simulink model "Gyro_Outage_Unit_Test"  (R2018b)
settings: Solver=VariableStepAuto  StartTime=0.0  StopTime=5600  FixedStep=fswParams.sample_time_s  RelTol=1e-8  AbsTol=1e-8
undefined symbols (not defined in the file or in its folder): B_eci_unit, Conversion_lib, DiscIntNeverNeededParam, e2sun_eci_unit, ECLIPSE, env_acc_mps2, Environment_lib, fswParams, gyro_body_radps, gyro_meas_valid, mag_body_T, mag_meas_valid, MEKF_Conversion_lib, MEKF_lib, photodiodes_A, q_body, r_eci_km, satelliteDynamics_lib, sc2sun_eci_unit, Sensors_Lib, simParams, solar_panel_power_W, sun_sensor_lib, sunsensor_2body_lib, sunsensor_body_deg, sunsensor_body_rad, sunsensor_valid, Triad, Triad_lib, v_eci_km, w_body_radps
libraries: aerolibutil x11, vrlib x10, sharedutil x8, simulink x5, dspmathops x4, sharedtransform x3, magnetometer_lib x3, gyroscope_lib x2, gravityGrad_Lib x1, atmoDrag_lib x1, magField_lib x1, solarPressure_lib x1
(part 1 of 3)
settings Model: Creator=kylle  LastModifiedBy=kylle

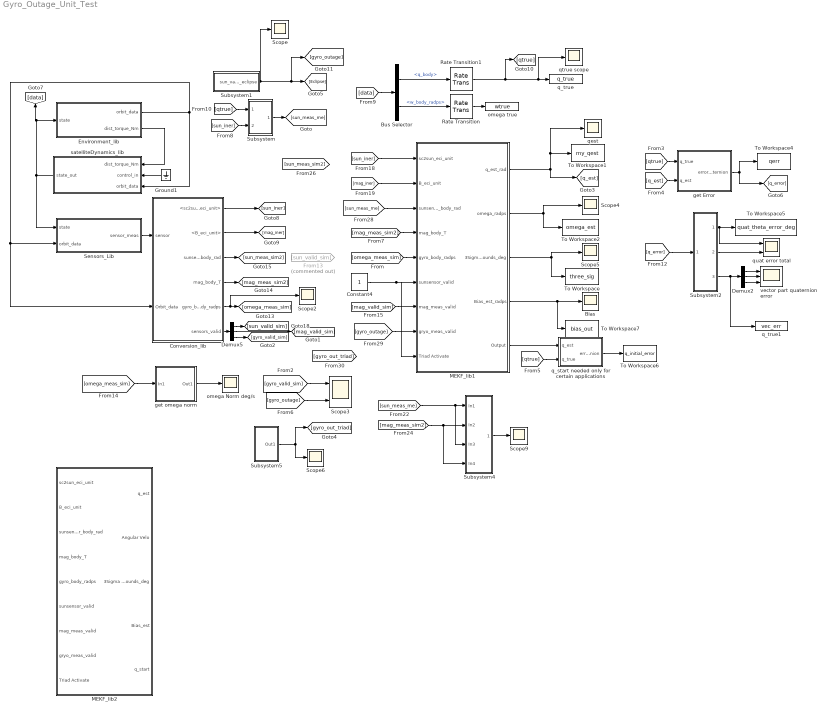
== system Gyro_Outage_Unit_Test ==
  Bias : Scope
  Bus Selector : BusSelector  OutputSignals=q_body,w_body_radps
  Constant4 : Constant
  Conversion_lib : Subsystem  AncestorBlock=MEKF_Conversion_lib/Conversion_lib
  Demux2 : Demux  Outputs=3
  Demux5 : Demux  Outputs=3
  Environment_lib : Subsystem  AncestorBlock=Environment_lib/Environment_lib
  From13 : From  Commented=on  GotoTag=sun_valid_sim
  Ground1 : Ground
  MEKF_lib1 : Subsystem  AncestorBlock=MEKF_lib/MEKF_lib
  MEKF_lib2 : Subsystem  AncestorBlock=MEKF_lib/MEKF_lib
  Rate Transition : RateTransition  InitialCondition=[0;0;0]  OutPortSampleTime=fswParams.sample_time_s
  Rate Transition1 : RateTransition  InitialCondition=[1;0;0;0]  OutPortSampleTime=fswParams.sample_time_s
  Scope{,2,4..6,9} (6 alike) : Scope
  Scope3 : Scope  NumInputPorts=2
  Sensors_Lib : Subsystem  AncestorBlock=Sensors_Lib/Sensors_Lib
  Subsystem : Subsystem
  Subsystem1 : Subsystem
  Subsystem2 : Subsystem
  Subsystem4 : Subsystem
  Subsystem5 : Subsystem
  To Workspace : ToWorkspace  VariableName=three_sig  SaveFormat=Timeseries  SampleTime=-1
  To Workspace1 : ToWorkspace  VariableName=my_qest  SaveFormat=Timeseries  SampleTime=-1
  To Workspace2 : ToWorkspace  VariableName=omega_est  SaveFormat=Timeseries  SampleTime=-1
  To Workspace4 : ToWorkspace  VariableName=qerr  SaveFormat=Timeseries  SampleTime=-1
  To Workspace5 : ToWorkspace  VariableName=quat_theta_error_deg  SaveFormat=Timeseries  SampleTime=-1
  To Workspace6 : ToWorkspace  VariableName=q_initial_error  SaveFormat=Timeseries  SampleTime=-1
  To Workspace7 : ToWorkspace  VariableName=bias_out  SaveFormat=Timeseries  SampleTime=-1
  get Error : Subsystem
  get omega norm : Subsystem
  omega Norm deg/s : Scope
  omega true : ToWorkspace  VariableName=wtrue  SaveFormat=Timeseries  SampleTime=-1
  q_start needed only for certain applications : Subsystem
  q_true : ToWorkspace  VariableName=q_true  SaveFormat=Timeseries  SampleTime=-1
  q_true1 : ToWorkspace  VariableName=vec_err  SaveFormat=Timeseries  SampleTime=-1
  qest : Scope
  "qtrue scope " : Scope
  quat error total : Scope  NumInputPorts=2
  satelliteDynamics_lib : Subsystem  AncestorBlock=satelliteDynamics_lib/satelliteDynamics_lib
  vector part quaternion error : Scope  NumInputPorts=3
  wires:
  get Error/1(error_quaternion) -> To Workspace4/1, [q_error]
  [q_est] -> get Error/2(q_est)
  [qtrue] -> get Error/1(q_true)
  Demux2/1 -> vector part quaternion error/1
  Demux2/2 -> vector part quaternion error/2
  Demux2/3 -> vector part quaternion error/3
  MEKF_lib1/1(q_est_rad) -> [q_est], qest/1, To Workspace1/1
  MEKF_lib1/2(omega_radps) -> To Workspace2/1, Scope4/1
  MEKF_lib1/3("3Sigma Bounds_deg ") -> Scope5/1, To Workspace/1
  MEKF_lib1/4(Bias_est_radps) -> Bias/1, To Workspace7/1
  Ground1/1 -> satelliteDynamics_lib/2(control_in)
  Environment_lib/1(orbit_data) -> satelliteDynamics_lib/3(orbit_data), Sensors_Lib/2(orbit_data), Conversion_lib/2(Orbit_data)
  Environment_lib/2(dist_torque_Nm) -> satelliteDynamics_lib/1(dist_torque_Nm)
  satelliteDynamics_lib/1(state_out) -> Environment_lib/1(state), [data], Sensors_Lib/1(state)
  Bus Selector/2 -> Rate Transition/1  "<w_body_radps>"
  [data] -> Bus Selector/1
  Bus Selector/1 -> Rate Transition1/1  "<q_body>"
  Sensors_Lib/1(sensor_meas) -> Conversion_lib/1(sensor)
  [mag_meas_sim2] -> MEKF_lib1/4(mag_body_T)
  [sun_iner] -> MEKF_lib1/1(sc2sun_eci_unit)
  [mag_iner] -> MEKF_lib1/2(B_eci_unit)
  [gyro_valid_sim] -> Scope3/1
  Conversion_lib/2(<B_eci_unit>) -> [mag_iner]
  Conversion_lib/1(<sc2sun_eci_unit>) -> [sun_iner]
  Conversion_lib/4(mag_body_T) -> [mag_meas_sim2]
  Conversion_lib/5(gyro_body_radps) -> Scope2/1, [omega_meas_sim]
  Demux5/2 -> [mag_valid_sim]
  Demux5/3 -> [gyro_valid_sim]
  Conversion_lib/6("sensors_valid ") -> Demux5/1
  q_start needed only for certain applications/1(error_quaternion) -> To Workspace6/1
  [qtrue] -> q_start needed only for certain applications/2(q_true)
  [qtrue] -> Subsystem/1(In1)
  [sun_iner] -> Subsystem/2(In2)
  Subsystem/1(Out1) -> [sun_meas_me]
  Conversion_lib/3(sunsensor_body_rad) -> [sun_meas_sim2]
  Demux5/1 -> [sun_valid_sim]
  Subsystem2/1(Out1) -> quat error total/1, To Workspace5/1
  [q_error] -> Subsystem2/1(In1)
  Subsystem2/2(Out2) -> quat error total/2
  Subsystem2/3(Out3) -> q_true1/1, Demux2/1
  Subsystem1/1(sun_valid_eclipse) -> Scope/1, [Eclipse], [gyro_outage]
  [omega_meas_sim] -> MEKF_lib1/5(gyro_body_radps)
  [mag_valid_sim] -> MEKF_lib1/7(mag_meas_valid)
  Rate Transition/1 -> omega true/1
  Rate Transition1/1 -> "qtrue scope "/1, q_true/1, [qtrue]
  [omega_meas_sim] -> get omega norm/1(In1)
  get omega norm/1(Out1) -> omega Norm deg/s/1
  [sun_meas_me] -> Subsystem4/3(In3), Subsystem4/1(In1)
  [mag_meas_sim2] -> Subsystem4/4(In4), Subsystem4/2(In2)
  Subsystem4/1(Out1) -> Scope9/1
  [sun_meas_me] -> MEKF_lib1/3(sunsensor_body_rad)
  Constant4/1 -> MEKF_lib1/9(Triad Activate), MEKF_lib1/6(sunsensor_valid)
  Subsystem5/1(Out1) -> [gyro_out_triad], Scope6/1
  [gyro_outage] -> MEKF_lib1/8(gryo_meas_valid)
  [gyro_outage] -> Scope3/2
  MEKF_lib1/5(Output) -> q_start needed only for certain applications/1(q_est)

== system Gyro_Outage_Unit_Test/Conversion_lib ==
  sensor : Inport
  Orbit_data : Inport  Port=2
  Bus Selector1 : BusSelector  OutputSignals=sc2sun_eci_unit,B_eci_unit
  Bus Selector2 : BusSelector  OutputSignals=sunsensor_body_deg,mag_body_T,gyro_body_radps,sunsensor_valid,mag_meas_valid,gyro_meas_valid
  Mux : Mux  Inputs=3
  Variable Selector : S-Function  AncestorBlock=dspindex/Variable Selector  FunctionName=sdspperm2  Parameters=1,NumInputs, rowsOrCols, IdxMode, Elements, FillMode, FillValues, errmode, 0, ZerOneIdxMode  SFunctionDeploymentMode=off  EnableBusSupport=off  mask(Variable Selector){NumInputs=1, rowsOrCols=Columns, IdxMode=Fixed, Elements=[1], ZerOneIdxMode=One-based, errmode=Clip Index, FillMode=off, FillValues=0, ShowPortLabels=off}
      mask prompts: NumInputs "Number of input signals:"; rowsOrCols "Select:"; IdxMode "Selector mode:"; ZerOneIdxMode "Index mode:"; errmode "Invalid index:"; FillMode "Fill empty spaces in outputs (for logical indexing)"; FillValues "Fill values:"; ShowPortLabels "Unused:"
      mask help:
      | Selects and/or reorders the rows or columns of the input according to a specified vector of indices (the indices need not be unique). The 'Selector mode' parameter determines whether the block uses the same indices for every input ('Fixed'), or uses different indices for every input ('Variable'). When set to 'Variable', you provide the vector of indices through an input port.
      |
      | When the indices are of Boolean data type the block performs logical indexing.
      mask init:
      | if ~isempty(NumInputs) && isfinite(NumInputs) && ~isnan(NumInputs) ...
      |  && isscalar(NumInputs) && isreal(NumInputs) && (NumInputs>0)
      |     maskdisplay = ['disp([''Select\n' get_param(gcbh, 'rowsOrCols') ''']);'];
      | 
      |     for i=1:NumInputs
      |         istr = int2str(i);
      |         maskdisplay = [maskdisplay 'port_label(''input'',' istr, ',''In' istr ''');'];
      |         maskdisplay = [maskdisplay 'port_label(''output'',' istr, ',''Out' istr ''');'];
      |     end
      | 
      |     if  IdxMode==2
      |         istr = int2str(NumInputs+1);
      |         maskdisplay = [maskdisplay 'port_label(''input'',' istr, ',''Idx'');'];
      |     end
      |     set_param(gcb, 'MaskDisplay', maskdisplay);
      | end
      mask Help: eval('blocksethelp');
      mask TypeOptions rowsOrCols: Rows | Columns
      mask TypeOptions IdxMode: Fixed | Variable
      mask Callback IdxMode: dspblkperm2;
      mask TypeOptions ZerOneIdxMode: Zero-based | One-based
      mask TypeOptions errmode: Clip Index | Clip and Warn | Generate Error
      mask Callback FillMode: dspblkperm2;
      mask Display: disp(['Select\nColumns']);port_label('input',1,'In1');port_label('output',1,'Out1');
  Variable Selector1 : S-Function  AncestorBlock=dspindex/Variable Selector  FunctionName=sdspperm2  Parameters=1,NumInputs, rowsOrCols, IdxMode, Elements, FillMode, FillValues, errmode, 0, ZerOneIdxMode  SFunctionDeploymentMode=off  EnableBusSupport=off  mask(Variable Selector){NumInputs=1, rowsOrCols=Columns, IdxMode=Fixed, Elements=[1], ZerOneIdxMode=One-based, errmode=Clip Index, FillMode=off, FillValues=0, ShowPortLabels=off}
      mask prompts: NumInputs "Number of input signals:"; rowsOrCols "Select:"; IdxMode "Selector mode:"; ZerOneIdxMode "Index mode:"; errmode "Invalid index:"; FillMode "Fill empty spaces in outputs (for logical indexing)"; FillValues "Fill values:"; ShowPortLabels "Unused:"
      mask help:
      | Selects and/or reorders the rows or columns of the input according to a specified vector of indices (the indices need not be unique). The 'Selector mode' parameter determines whether the block uses the same indices for every input ('Fixed'), or uses different indices for every input ('Variable'). When set to 'Variable', you provide the vector of indices through an input port.
      |
      | When the indices are of Boolean data type the block performs logical indexing.
      mask init: same as Gyro_Outage_Unit_Test/Conversion_lib/Variable Selector
      mask Help: eval('blocksethelp');
      mask TypeOptions rowsOrCols: Rows | Columns
      mask TypeOptions IdxMode: Fixed | Variable
      mask Callback IdxMode: dspblkperm2;
      mask TypeOptions ZerOneIdxMode: Zero-based | One-based
      mask TypeOptions errmode: Clip Index | Clip and Warn | Generate Error
      mask Callback FillMode: dspblkperm2;
      mask Display: disp(['Select\nColumns']);port_label('input',1,'In1');port_label('output',1,'Out1');
  Variable Selector2 : S-Function  AncestorBlock=dspindex/Variable Selector  FunctionName=sdspperm2  Parameters=1,NumInputs, rowsOrCols, IdxMode, Elements, FillMode, FillValues, errmode, 0, ZerOneIdxMode  SFunctionDeploymentMode=off  EnableBusSupport=off  mask(Variable Selector){NumInputs=1, rowsOrCols=Rows, IdxMode=Fixed, Elements=[1], ZerOneIdxMode=One-based, errmode=Clip Index, FillMode=off, FillValues=0, ShowPortLabels=off}
      mask prompts: NumInputs "Number of input signals:"; rowsOrCols "Select:"; IdxMode "Selector mode:"; ZerOneIdxMode "Index mode:"; errmode "Invalid index:"; FillMode "Fill empty spaces in outputs (for logical indexing)"; FillValues "Fill values:"; ShowPortLabels "Unused:"
      mask help:
      | Selects and/or reorders the rows or columns of the input according to a specified vector of indices (the indices need not be unique). The 'Selector mode' parameter determines whether the block uses the same indices for every input ('Fixed'), or uses different indices for every input ('Variable'). When set to 'Variable', you provide the vector of indices through an input port.
      |
      | When the indices are of Boolean data type the block performs logical indexing.
      mask init: same as Gyro_Outage_Unit_Test/Conversion_lib/Variable Selector
      mask Help: eval('blocksethelp');
      mask TypeOptions rowsOrCols: Rows | Columns
      mask TypeOptions IdxMode: Fixed | Variable
      mask Callback IdxMode: dspblkperm2;
      mask TypeOptions ZerOneIdxMode: Zero-based | One-based
      mask TypeOptions errmode: Clip Index | Clip and Warn | Generate Error
      mask Callback FillMode: dspblkperm2;
      mask Display: disp(['Select\nRows']);port_label('input',1,'In1');port_label('output',1,'Out1');
  Variable Selector3 : S-Function  AncestorBlock=dspindex/Variable Selector  FunctionName=sdspperm2  Parameters=1,NumInputs, rowsOrCols, IdxMode, Elements, FillMode, FillValues, errmode, 0, ZerOneIdxMode  SFunctionDeploymentMode=off  EnableBusSupport=off  mask(Variable Selector){NumInputs=1, rowsOrCols=Rows, IdxMode=Fixed, Elements=[1], ZerOneIdxMode=One-based, errmode=Clip Index, FillMode=off, FillValues=0, ShowPortLabels=off}
      mask prompts: NumInputs "Number of input signals:"; rowsOrCols "Select:"; IdxMode "Selector mode:"; ZerOneIdxMode "Index mode:"; errmode "Invalid index:"; FillMode "Fill empty spaces in outputs (for logical indexing)"; FillValues "Fill values:"; ShowPortLabels "Unused:"
      mask help:
      | Selects and/or reorders the rows or columns of the input according to a specified vector of indices (the indices need not be unique). The 'Selector mode' parameter determines whether the block uses the same indices for every input ('Fixed'), or uses different indices for every input ('Variable'). When set to 'Variable', you provide the vector of indices through an input port.
      |
      | When the indices are of Boolean data type the block performs logical indexing.
      mask init: same as Gyro_Outage_Unit_Test/Conversion_lib/Variable Selector
      mask Help: eval('blocksethelp');
      mask TypeOptions rowsOrCols: Rows | Columns
      mask TypeOptions IdxMode: Fixed | Variable
      mask Callback IdxMode: dspblkperm2;
      mask TypeOptions ZerOneIdxMode: Zero-based | One-based
      mask TypeOptions errmode: Clip Index | Clip and Warn | Generate Error
      mask Callback FillMode: dspblkperm2;
      mask Display: disp(['Select\nRows']);port_label('input',1,'In1');port_label('output',1,'Out1');
  sunsensor_body_rad1 : Subsystem  AncestorBlock=sunsensor_2body_lib/sunsensor_body_rad
  <sc2sun_eci_unit> : Outport
  <B_eci_unit> : Outport  Port=2
  sunsensor_body_rad : Outport  Port=3
  mag_body_T : Outport  Port=4
  gyro_body_radps : Outport  Port=5
  "sensors_valid " : Outport  Port=6
  wires:
  Bus Selector2/3 -> Variable Selector/1  "<gyro_body_radps>"
  Bus Selector1/2 -> <B_eci_unit>/1  "<B_eci_unit>"
  Bus Selector2/1 -> sunsensor_body_rad1/1(<sunsensor_body_deg>)  "<sunsensor_body_deg>"
  Bus Selector2/2 -> Variable Selector1/1  "<mag_body_T>"
  sunsensor_body_rad1/1(Out1) -> sunsensor_body_rad/1
  Bus Selector2/5 -> Variable Selector3/1  "<mag_meas_valid>"
  Bus Selector2/6 -> Variable Selector2/1  "<gyro_meas_valid>"
  sensor/1 -> Bus Selector2/1
  Variable Selector1/1 -> mag_body_T/1
  Bus Selector1/1 -> <sc2sun_eci_unit>/1  "<sc2sun_eci_unit>"
  Orbit_data/1 -> Bus Selector1/1
  Variable Selector/1 -> gyro_body_radps/1
  Variable Selector2/1 -> Mux/3
  Variable Selector3/1 -> Mux/2
  Bus Selector2/4 -> Mux/1  "<sunsensor_valid>"
  Mux/1 -> "sensors_valid "/1

== system Gyro_Outage_Unit_Test/Environment_lib ==
  state : Inport
  Bus Assignment : BusAssignment  AssignedSignals=env_acc_mps2,e2sun_eci_unit,sc2sun_eci_unit,ECLIPSE,B_eci_unit
  Disturbances : Subsystem
  Terminator{1..2,5,8..9,11..16} (11 alike) : Terminator
  clock_lib : clock_lib/clock_lib  SystemSampleTime=-1
  orbit_data_bus : orbit_data_bus/orbit_data_bus  SystemSampleTime=-1
  "time_lib " : time_Lib/time_lib    SystemSampleTime=-1
  orbit_data : Outport
  dist_torque_Nm : Outport  Port=2
  wires:
  Bus Assignment/1 -> orbit_data/1
  orbit_data_bus/1 -> Bus Assignment/1
  "time_lib "/10 -> Terminator2/1
  state/1 -> Disturbances/1(state)
  Disturbances/1(env_acc_mps2) -> Bus Assignment/2
  Disturbances/4(ECLIPSE) -> Bus Assignment/5
  "time_lib "/9 -> Terminator13/1
  [ymdhms_utc] -> Disturbances/5(ymdhms_utc)
  "time_lib "/7 -> Terminator11/1
  "time_lib "/11 -> Terminator14/1
  "time_lib "/8 -> Terminator12/1
  "time_lib "/1 -> Terminator5/1
  Disturbances/6(dist_torque_Nm) -> dist_torque_Nm/1
  clock_lib/1 -> "time_lib "/1, [MET_utc_s]
  "time_lib "/5 -> Terminator9/1
  "time_lib "/14 -> [eci2ecef]
  [eci2ecef] -> Disturbances/3(eci2ecef)
  "time_lib "/3 -> [ymdhms_utc]
  "time_lib "/6 -> [MET_ut1_jc]
  "time_lib "/12 -> Terminator15/1
  Disturbances/3(sc2sun_eci_unit) -> Bus Assignment/4
  [MET_ut1_jc] -> Disturbances/2(time_ut1_jc)
  "time_lib "/2 -> Terminator1/1
  "time_lib "/13 -> Terminator16/1
  "time_lib "/4 -> Terminator8/1
  Disturbances/2(e2sun_eci_unit) -> Bus Assignment/3
  Disturbances/5(B_eci_T) -> Bus Assignment/6
  [MET_utc_s] -> Disturbances/4(utc_s)

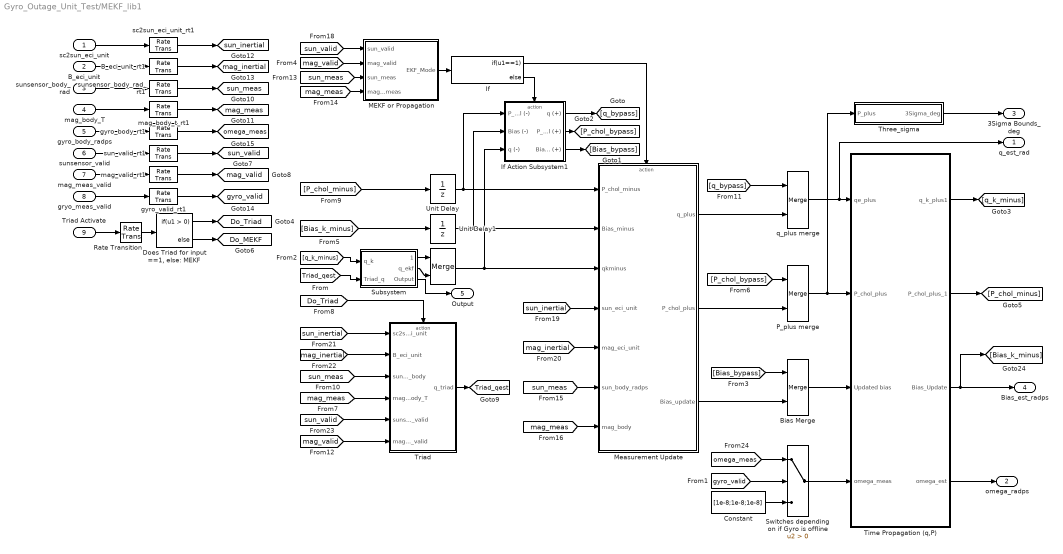
== system Gyro_Outage_Unit_Test/MEKF_lib1 ==
  sc2sun_eci_unit : Inport
  B_eci_unit : Inport  Port=2
  sunsensor_body_rad : Inport  Port=3
  mag_body_T : Inport  Port=4
  gyro_body_radps : Inport  Port=5
  sunsensor_valid : Inport  Port=6
  mag_meas_valid : Inport  Port=7
  gryo_meas_valid : Inport  Port=8
  Triad Activate : Inport  Port=9
  " " : Merge
  B_eci_unit_rt1 : RateTransition  InitialCondition=fswParams.estimation.ic.B_eci_unit_rt  OutPortSampleTime=fswParams.sample_time_s
  Bias Merge : Merge
  Constant : Constant  Value=[1e-8;1e-8;1e-8]
  "Does Triad for input ==1, else: MEKF" : If
  If : If  IfExpression=u1==1
  If Action Subsystem1 : Subsystem  TreatAsAtomicUnit=on
  MEKF or Propagation : Subsystem
  Measurement Update : Subsystem  TreatAsAtomicUnit=on
  P_plus merge : Merge
  Rate Transition : RateTransition  OutPortSampleTime=fswParams.sample_time_s
  Subsystem : Subsystem
  "Switches depending on if Gyro is offline " : Switch  Criteria=u2 > Threshold
  Three_sigma : Subsystem
  Time Propagation (q,P) : Subsystem
  Triad : Subsystem  TreatAsAtomicUnit=on
  Unit Delay : UnitDelay  InitialCondition=fswParams.estimation.ic.Pchol_init  SampleTime=fswParams.sample_time_s
  Unit Delay1 : UnitDelay  InitialCondition=fswParams.estimation.ic.Beta_init  SampleTime=fswParams.sample_time_s
  gyro_body_rt1 : RateTransition  InitialCondition=fswParams.estimation.ic.gyro_meas_rt  OutPortSampleTime=fswParams.sample_time_s
  gyro_valid_rt1 : RateTransition  InitialCondition=fswParams.estimation.ic.gyro_valid_rt  OutPortSampleTime=fswParams.sample_time_s
  mag_body_t_rt1 : RateTransition  InitialCondition=fswParams.estimation.ic.mag_body_rt  OutPortSampleTime=fswParams.sample_time_s
  mag_valid_rt1 : RateTransition  InitialCondition=fswParams.estimation.ic.mag_valid_rt  OutPortSampleTime=fswParams.sample_time_s
  q_plus merge : Merge
  sc2sun_eci_unit_rt1 : RateTransition  InitialCondition=fswParams.estimation.ic.sc2sun_eci_unit_rt  OutPortSampleTime=fswParams.sample_time_s
  sun_valid_rt1 : RateTransition  InitialCondition=fswParams.estimation.ic.sun_valid_rt  OutPortSampleTime=fswParams.sample_time_s
  sunsensor_body_rad_rt1 : RateTransition  InitialCondition=fswParams.estimation.ic.sunsensor_body_rad_rt  OutPortSampleTime=fswParams.sample_time_s
  q_est_rad : Outport
  omega_radps : Outport  Port=2
  "3Sigma Bounds_deg " : Outport  Port=3
  Bias_est_radps : Outport  Port=4
  Output : Outport  Port=5
  tag scope: Do_MEKF=global, Do_Triad=global, Triad_qest=global, gyro_valid=global, mag_inertial=global, mag_meas=global, mag_valid=global, omega_meas=global, sun_inertial=global, sun_meas=global, sun_valid=global
  wires:
  q_plus merge/1 -> q_est_rad/1, Time Propagation (q,P)/1(qe_plus)
  Time Propagation (q,P)/4(omega_est) -> omega_radps/1
  Three_sigma/1(3Sigma_deg) -> "3Sigma Bounds_deg "/1
  Time Propagation (q,P)/3(Bias_Update) -> Bias_est_radps/1, [Bias_k_minus]
  Measurement Update/2(P_chol_plus) -> P_plus merge/2
  [P_chol_bypass] -> P_plus merge/1
  P_plus merge/1 -> Three_sigma/1(P_plus), Time Propagation (q,P)/2(P_chol_plus)
  Constant/1 -> "Switches depending on if Gyro is offline "/3
  gryo_meas_valid/1 -> gyro_valid_rt1/1
  Bias Merge/1 -> Time Propagation (q,P)/3(Updated bias)
  If Action Subsystem1/3(Bias (+)) -> [Bias_bypass]
  If Action Subsystem1/2(P_chol (+)) -> [P_chol_bypass]
  [Bias_bypass] -> Bias Merge/1
  [q_bypass] -> q_plus merge/1
  If Action Subsystem1/1(q (+)) -> [q_bypass]
  "Switches depending on if Gyro is offline "/1 -> Time Propagation (q,P)/4(omega_meas)
  Measurement Update/3(Bias_update) -> Bias Merge/2
  Measurement Update/1(q_plus) -> q_plus merge/2
  [P_chol_minus] -> Unit Delay/1
  [Bias_k_minus] -> Unit Delay1/1
  If/2 -> If Action Subsystem1/Action
  If/1 -> Measurement Update/Action
  Time Propagation (q,P)/2(P_chol_plus_1) -> [P_chol_minus]
  Time Propagation (q,P)/1(q_k_plus1) -> [q_k_minus]
  sc2sun_eci_unit/1 -> sc2sun_eci_unit_rt1/1
  B_eci_unit/1 -> B_eci_unit_rt1/1
  mag_body_T/1 -> mag_body_t_rt1/1
  sunsensor_body_rad/1 -> sunsensor_body_rad_rt1/1
  Rate Transition/1 -> "Does Triad for input ==1, else: MEKF"/1
  Triad Activate/1 -> Rate Transition/1
  "Does Triad for input ==1, else: MEKF"/1 -> [Do_Triad]
  "Does Triad for input ==1, else: MEKF"/2 -> [Do_MEKF]
  sunsensor_valid/1 -> sun_valid_rt1/1
  mag_meas_valid/1 -> mag_valid_rt1/1
  gyro_body_radps/1 -> gyro_body_rt1/1
  [sun_meas] -> Measurement Update/6(sun_body_radps)
  sunsensor_body_rad_rt1/1 -> [sun_meas]
  mag_body_t_rt1/1 -> [mag_meas]
  [mag_meas] -> Measurement Update/7(mag_body)
  sun_valid_rt1/1 -> [sun_valid]
  mag_valid_rt1/1 -> [mag_valid]
  Unit Delay/1 -> If Action Subsystem1/1(P_chol (-)), Measurement Update/1(P_chol_minus)
  Unit Delay1/1 -> If Action Subsystem1/2(Bias (-)), Measurement Update/2(Bias_minus)
  " "/1 -> If Action Subsystem1/3(q (-)), Measurement Update/3(qkminus)
  MEKF or Propagation/1(EKF_Mode) -> If/1
  sc2sun_eci_unit_rt1/1 -> [sun_inertial]
  B_eci_unit_rt1/1 -> [mag_inertial]
  gyro_valid_rt1/1 -> [gyro_valid]
  gyro_body_rt1/1 -> [omega_meas]
  [omega_meas] -> "Switches depending on if Gyro is offline "/1
  [mag_inertial] -> Measurement Update/5(mag_eci_unit)
  [sun_inertial] -> Measurement Update/4(sun_eci_unit)
  Triad/1(q_triad) -> [Triad_qest]
  [q_k_minus] -> Subsystem/1(q_k)
  Subsystem/1(Triad_qest) -> " "/1
  Subsystem/2(q_ekf) -> " "/2
  [Triad_qest] -> Subsystem/2(Triad_q)
  [gyro_valid] -> "Switches depending on if Gyro is offline "/2
  [sun_valid] -> MEKF or Propagation/1(sun_valid)
  [mag_valid] -> MEKF or Propagation/2(mag_valid)
  [sun_meas] -> MEKF or Propagation/3(sun_meas)
  [mag_meas] -> MEKF or Propagation/4(mag_meas)
  [sun_meas] -> Triad/3(sun_meas_rad_body)
  [Do_Triad] -> Triad/Action
  [sun_valid] -> Triad/5(sunsensor_valid)
  [mag_meas] -> Triad/4(mag_meas_body_T)
  [sun_inertial] -> Triad/1(sc2sun_eci_unit)
  [mag_valid] -> Triad/6(magsensor_valid)
  [mag_inertial] -> Triad/2(B_eci_unit)
  Subsystem/3(Output) -> Output/1

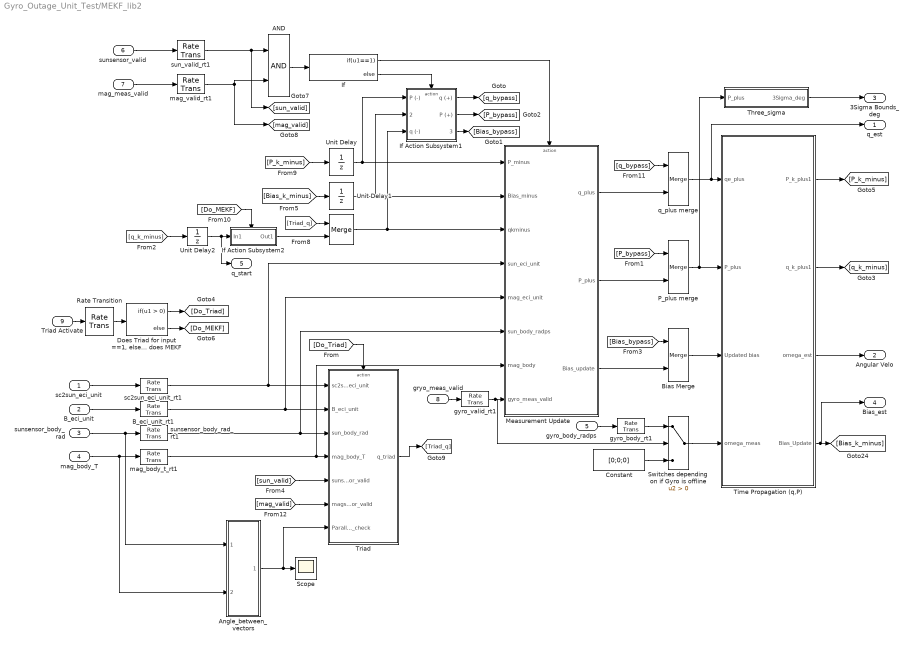
== system Gyro_Outage_Unit_Test/MEKF_lib2 ==
  sc2sun_eci_unit : Inport
  B_eci_unit : Inport  Port=2
  sunsensor_body_rad : Inport  Port=3
  mag_body_T : Inport  Port=4
  gyro_body_radps : Inport  Port=5
  sunsensor_valid : Inport  Port=6
  mag_meas_valid : Inport  Port=7
  gryo_meas_valid : Inport  Port=8
  Triad Activate : Inport  Port=9
  " " : Merge
  AND : Logic  AllPortsSameDT=off  OutDataTypeStr=boolean
  Angle_between_vectors : Subsystem
  B_eci_unit_rt1 : RateTransition  InitialCondition=fswParams.estimation.ic.B_eci_unit_rt  OutPortSampleTime=fswParams.sample_time_s
  Bias Merge : Merge
  Constant : Constant  Value=[0;0;0]
  "Does Triad for input ==1, else does MEKF" : If
  If : If  IfExpression=u1==1
  If Action Subsystem1 : Subsystem  TreatAsAtomicUnit=on
  If Action Subsystem2 : Subsystem  TreatAsAtomicUnit=on
  Measurement Update : Subsystem  TreatAsAtomicUnit=on
  P_plus merge : Merge
  Rate Transition : RateTransition  OutPortSampleTime=fswParams.sample_time_s
  Scope : Scope
  "Switches depending on if Gyro is offline " : Switch  Criteria=u2 > Threshold
  Three_sigma : Subsystem
  Time Propagation (q,P) : Subsystem  AncestorBlock=MEKF_Library/Multiplicative Extended Kalman Filter/TIME PROPAGATION of Q_EST, COVARIANCE
  Triad : Subsystem  AncestorBlock=Triad_lib/Triad  TreatAsAtomicUnit=on
  Unit Delay : UnitDelay  InitialCondition=fswParams.estimation.ic.Pchol_init  SampleTime=fswParams.sample_time_s
  Unit Delay1 : UnitDelay  InitialCondition=fswParams.estimation.ic.Beta_init  SampleTime=fswParams.sample_time_s
  Unit Delay2 : UnitDelay  InitialCondition=[0;0.707106781186547;0.707106781186547;0]  SampleTime=fswParams.sample_time_s
  gyro_body_rt1 : RateTransition  InitialCondition=fswParams.estimation.ic.gyro_meas_rt  OutPortSampleTime=fswParams.sample_time_s
  gyro_valid_rt1 : RateTransition  InitialCondition=fswParams.estimation.ic.gyro_valid_rt  OutPortSampleTime=fswParams.sample_time_s
  mag_body_t_rt1 : RateTransition  InitialCondition=fswParams.estimation.ic.mag_body_rt  OutPortSampleTime=fswParams.sample_time_s
  mag_valid_rt1 : RateTransition  InitialCondition=fswParams.estimation.ic.mag_valid_rt  OutPortSampleTime=fswParams.sample_time_s
  q_plus merge : Merge
  sc2sun_eci_unit_rt1 : RateTransition  InitialCondition=fswParams.estimation.ic.sc2sun_eci_unit_rt  OutPortSampleTime=fswParams.sample_time_s
  sun_valid_rt1 : RateTransition  InitialCondition=fswParams.estimation.ic.sun_valid_rt  OutPortSampleTime=fswParams.sample_time_s
  sunsensor_body_rad_rt1 : RateTransition  InitialCondition=fswParams.estimation.ic.sunsensor_body_rad_rt  OutPortSampleTime=fswParams.sample_time_s
  q_est : Outport
  "Angular Velo " : Outport  Port=2
  "3Sigma Bounds_deg " : Outport  Port=3
  Bias_est : Outport  Port=4
  q_start : Outport  Port=5
  wires:
  AND/1 -> If/1
  "Does Triad for input ==1, else does MEKF"/2 -> [Do_MEKF]
  "Does Triad for input ==1, else does MEKF"/1 -> [Do_Triad]
  Triad Activate/1 -> Rate Transition/1
  Rate Transition/1 -> "Does Triad for input ==1, else does MEKF"/1
  Triad/1(q_triad) -> [Triad_q]
  [Do_Triad] -> Triad/Action
  If Action Subsystem2/1(Out1) -> " "/2
  [Triad_q] -> " "/1
  [q_k_minus] -> Unit Delay2/1
  Unit Delay2/1 -> q_start/1, If Action Subsystem2/1(In1)
  [Do_MEKF] -> If Action Subsystem2/Action
  [mag_valid] -> Triad/6(magsensor_valid)
  [sun_valid] -> Triad/5(sunsensor_valid)
  " "/1 -> If Action Subsystem1/3(q (-)), Measurement Update/3(qkminus)
  Unit Delay/1 -> Measurement Update/1(P_minus), If Action Subsystem1/1(P (-))
  Unit Delay1/1 -> Measurement Update/2(Bias_minus), If Action Subsystem1/2(Bias (-))
  Time Propagation (q,P)/2(q_k_plus1) -> [q_k_minus]
  Time Propagation (q,P)/1(P_k_plus1) -> [P_k_minus]
  If/1 -> Measurement Update/Action
  If/2 -> If Action Subsystem1/Action
  [Bias_k_minus] -> Unit Delay1/1
  [P_k_minus] -> Unit Delay/1
  Measurement Update/1(q_plus) -> q_plus merge/2
  Measurement Update/3(Bias_update) -> Bias Merge/2
  "Switches depending on if Gyro is offline "/1 -> Time Propagation (q,P)/4(omega_meas)
  If Action Subsystem1/1(q (+)) -> [q_bypass]
  [Bias_bypass] -> Bias Merge/1
  If Action Subsystem1/2(P (+)) -> [P_bypass]
  If Action Subsystem1/3(Bias (+)) -> [Bias_bypass]
  Bias Merge/1 -> Time Propagation (q,P)/3(Updated bias)
  P_plus merge/1 -> Time Propagation (q,P)/2(P_plus), Three_sigma/1(P_plus)
  [P_bypass] -> P_plus merge/1
  Measurement Update/2(P_plus) -> P_plus merge/2
  Time Propagation (q,P)/4(Bias_Update) -> [Bias_k_minus], Bias_est/1
  Three_sigma/1(3Sigma_deg) -> "3Sigma Bounds_deg "/1
  Time Propagation (q,P)/3(omega_est) -> "Angular Velo "/1
  q_plus merge/1 -> Time Propagation (q,P)/1(qe_plus), q_est/1
  sunsensor_valid/1 -> sun_valid_rt1/1
  mag_meas_valid/1 -> mag_valid_rt1/1
  sc2sun_eci_unit/1 -> sc2sun_eci_unit_rt1/1
  B_eci_unit/1 -> B_eci_unit_rt1/1
  sunsensor_body_rad/1 -> Angle_between_vectors/1(sun_meas_rad_body), sunsensor_body_rad_rt1/1
  mag_body_T/1 -> Angle_between_vectors/2(mag_meas_T_body), mag_body_t_rt1/1
  gryo_meas_valid/1 -> gyro_valid_rt1/1
  gyro_body_radps/1 -> gyro_body_rt1/1
  B_eci_unit_rt1/1 -> Triad/2(B_eci_unit), Measurement Update/5(mag_eci_unit)
  mag_body_t_rt1/1 -> Measurement Update/7(mag_body), Triad/4(mag_body_T)
  sc2sun_eci_unit_rt1/1 -> Triad/1(sc2sun_eci_unit), Measurement Update/4(sun_eci_unit)
  sunsensor_body_rad_rt1/1 -> Triad/3(sun_body_rad), Measurement Update/6(sun_body_radps)
  gyro_body_rt1/1 -> "Switches depending on if Gyro is offline "/1
  gyro_valid_rt1/1 -> "Switches depending on if Gyro is offline "/2, Measurement Update/8(gyro_meas_valid)
  mag_valid_rt1/1 -> AND/2, [mag_valid]
  sun_valid_rt1/1 -> [sun_valid], AND/1
  [q_bypass] -> q_plus merge/1
  Constant/1 -> "Switches depending on if Gyro is offline "/3
  Angle_between_vectors/1(Out1) -> Triad/7(Parallel_meas_check), Scope/1

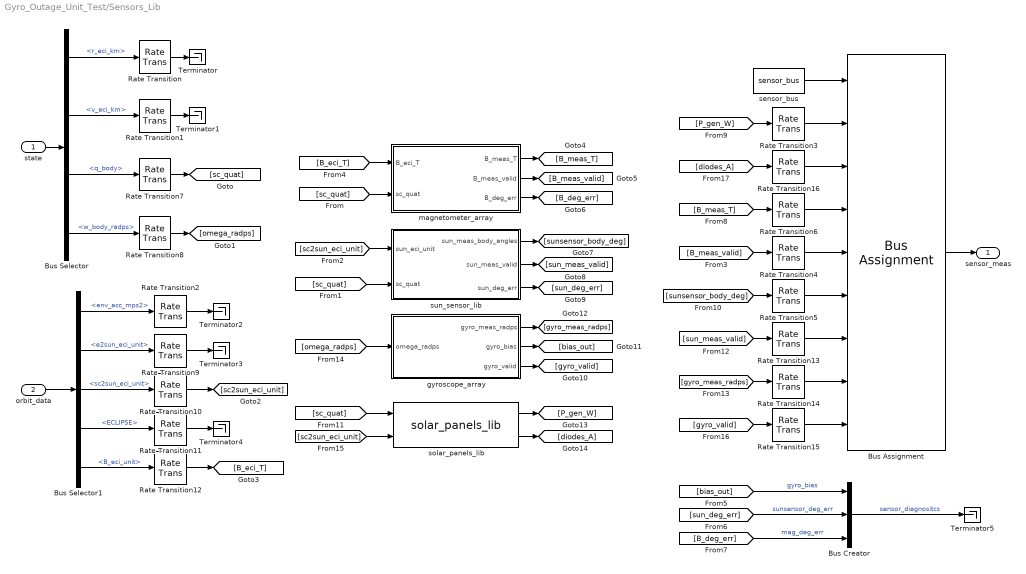
== system Gyro_Outage_Unit_Test/Sensors_Lib ==
  state : Inport
  orbit_data : Inport  Port=2
  Bus Assignment : BusAssignment  AssignedSignals=solar_panel_power_W,photodiodes_A,mag_body_T,mag_meas_valid,sunsensor_body_deg,sunsensor_valid,gyro_body_radps,gyro_meas_valid
  Bus Creator : BusCreator  Inputs=3
  Bus Selector : BusSelector  OutputSignals=r_eci_km,v_eci_km,q_body,w_body_radps
  Bus Selector1 : BusSelector  OutputSignals=env_acc_mps2,e2sun_eci_unit,sc2sun_eci_unit,ECLIPSE,B_eci_unit
  Rate Transition{,1..16} (17 alike) : RateTransition  OutPortSampleTime=simParams.sensors.sample_time_s
  Terminator{,1..5} (6 alike) : Terminator
  gyroscope_array : Subsystem
  magnetometer_array : Subsystem
  sensor_bus : sensor_bus/sensor_bus  SystemSampleTime=-1
  solar_panels_lib : solar_panels_lib/solar_panels_lib  SystemSampleTime=-1
  "sun_sensor_lib " : Subsystem  AncestorBlock=sun_sensor_lib/sun_sensor_lib
  sensor_meas : Outport
  wires:
  state/1 -> Bus Selector/1
  [diodes_A] -> Rate Transition16/1
  Rate Transition16/1 -> Bus Assignment/3
  Rate Transition3/1 -> Bus Assignment/2
  Rate Transition6/1 -> Bus Assignment/4
  Rate Transition4/1 -> Bus Assignment/5
  Rate Transition5/1 -> Bus Assignment/6
  Rate Transition13/1 -> Bus Assignment/7
  Rate Transition14/1 -> Bus Assignment/8
  Rate Transition15/1 -> Bus Assignment/9
  solar_panels_lib/2 -> [diodes_A]
  Bus Creator/1 -> Terminator5/1  "sensor_diagnositcs"
  [B_deg_err] -> Bus Creator/3  "mag_deg_err"
  [sun_deg_err] -> Bus Creator/2  "sunsensor_deg_err"
  [bias_out] -> Bus Creator/1  "gyro_bias"
  [gyro_valid] -> Rate Transition15/1
  [gyro_meas_radps] -> Rate Transition14/1
  [sun_meas_valid] -> Rate Transition13/1
  [sunsensor_body_deg] -> Rate Transition5/1
  [B_meas_valid] -> Rate Transition4/1
  [P_gen_W] -> Rate Transition3/1
  [B_meas_T] -> Rate Transition6/1
  solar_panels_lib/1 -> [P_gen_W]
  [sc_quat] -> solar_panels_lib/1
  [sc2sun_eci_unit] -> solar_panels_lib/2
  Bus Selector1/1 -> Rate Transition2/1  "<env_acc_mps2>"
  Rate Transition2/1 -> Terminator2/1
  Rate Transition9/1 -> Terminator3/1
  Bus Selector1/2 -> Rate Transition9/1  "<e2sun_eci_unit>"
  Rate Transition10/1 -> [sc2sun_eci_unit]
  Bus Selector1/3 -> Rate Transition10/1  "<sc2sun_eci_unit>"
  Rate Transition11/1 -> Terminator4/1
  Bus Selector1/4 -> Rate Transition11/1  "<ECLIPSE>"
  Rate Transition12/1 -> [B_eci_T]
  Bus Selector1/5 -> Rate Transition12/1  "<B_eci_unit>"
  Rate Transition/1 -> Terminator/1
  Bus Selector/1 -> Rate Transition/1  "<r_eci_km>"
  Rate Transition1/1 -> Terminator1/1
  Rate Transition7/1 -> [sc_quat]
  Bus Selector/3 -> Rate Transition7/1  "<q_body>"
  Rate Transition8/1 -> [omega_radps]
  gyroscope_array/3(gyro_valid) -> [gyro_valid]
  gyroscope_array/2(gyro_bias) -> [bias_out]
  gyroscope_array/1(gyro_meas_radps) -> [gyro_meas_radps]
  "sun_sensor_lib "/3(sun_deg_err) -> [sun_deg_err]
  "sun_sensor_lib "/2(sun_meas_valid) -> [sun_meas_valid]
  "sun_sensor_lib "/1(sun_meas_body_angles) -> [sunsensor_body_deg]
  magnetometer_array/3(B_deg_err) -> [B_deg_err]
  magnetometer_array/2(B_meas_valid) -> [B_meas_valid]
  magnetometer_array/1(B_meas_T) -> [B_meas_T]
  sensor_bus/1 -> Bus Assignment/1
  [B_eci_T] -> magnetometer_array/1(B_eci_T)
  [sc2sun_eci_unit] -> "sun_sensor_lib "/1(sun_eci_unit)
  orbit_data/1 -> Bus Selector1/1
  [omega_radps] -> gyroscope_array/1(omega_radps)
  [sc_quat] -> "sun_sensor_lib "/2(sc_quat)
  [sc_quat] -> magnetometer_array/2(sc_quat)
  Bus Assignment/1 -> sensor_meas/1
  Bus Selector/4 -> Rate Transition8/1  "<w_body_radps>"
  Bus Selector/2 -> Rate Transition1/1  "<v_eci_km>"

== system Gyro_Outage_Unit_Test/Subsystem ==
  In1 : Inport
  In2 : Inport  Port=2
  Add1 : Sum
  Gain2 : Gain  Gain=0.5/(sqrt(2)*3.0)*pi/180
  Matrix Multiply : Product  Multiplication=Matrix(*)
  Quaternions to Direction Cosine Matrix : sharedtransform/Quaternions to  Direction Cosine Matrix  aMode=aMode
      settings: SourceProductName=Aerospace Blockset  SourceProductBaseCode=AE
  Random Number : RandomNumber  Variance=[1;1;1]  SampleTime=0.1
  Out1 : Outport
  wires:
  Quaternions to Direction Cosine Matrix/1 -> Matrix Multiply/1
  In1/1 -> Quaternions to Direction Cosine Matrix/1
  Add1/1 -> Out1/1
  Random Number/1 -> Gain2/1
  Gain2/1 -> Add1/1
  In2/1 -> Matrix Multiply/2
  Matrix Multiply/1 -> Add1/2

== system Gyro_Outage_Unit_Test/Subsystem1 ==
  Add : Sum  Inputs=+++
  Eclipse_end : Step  Time=3700.1  SampleTime=0
  Eclipse_time : Step  Tag=Eclipse_time  Time=1900  After=-1  SampleTime=0
  Scope1 : Scope
  Step : Step  Time=0  SampleTime=0
  sun_valid_eclipse : Outport
  wires:
  Eclipse_end/1 -> Add/3
  Add/1 -> sun_valid_eclipse/1, Scope1/1
  Step/1 -> Add/1
  Eclipse_time/1 -> Add/2

== system Gyro_Outage_Unit_Test/Subsystem2 ==
  In1 : Inport
  Acos : Trigonometry  Operator=acos
  Demux3 : Demux
  Gain1 : Gain  Gain=180/pi
  Gain6 : Gain  Gain=2*180/pi
  Mux : Mux  Inputs=3
  Out1 : Outport
  Out2 : Outport  Port=2
  Out3 : Outport  Port=3
  wires:
  Acos/1 -> Gain6/1
  Mux/1 -> Gain1/1
  Demux3/4 -> Mux/3
  Demux3/2 -> Mux/1
  Demux3/3 -> Mux/2
  Gain1/1 -> Out3/1
  Demux3/1 -> Acos/1
  Gain6/1 -> Out1/1
  In1/1 -> Demux3/1
  [sun_valid_sim] -> Out2/1

== system Gyro_Outage_Unit_Test/Subsystem4 ==
  In1 : Inport
  In2 : Inport  Port=2
  In3 : Inport  Port=3
  In4 : Inport  Port=4
  Acos : Trigonometry  Operator=acos
  Divide : Product  Inputs=*/
  Dot Product : DotProduct  InputSameDT=on  OutDataTypeStr=Inherit: Inherit via internal rule
  Dot Product1 : DotProduct  InputSameDT=on  OutDataTypeStr=Inherit: Inherit via internal rule
  Dot Product2 : DotProduct  InputSameDT=on  OutDataTypeStr=Inherit: Inherit via internal rule
  Gain : Gain  Gain=180/pi
  Multiply : Product
  Scope : Scope
  Sqrt : Sqrt  SaturateOnIntegerOverflow=on
  Sqrt1 : Sqrt  SaturateOnIntegerOverflow=on
  Out1 : Outport
  wires:
  Dot Product1/1 -> Sqrt/1
  Divide/1 -> Scope/1, Acos/1
  Acos/1 -> Gain/1
  In2/1 -> Dot Product/2
  In3/1 -> Dot Product1/2, Dot Product1/1
  In4/1 -> Dot Product2/2, Dot Product2/1
  Sqrt1/1 -> Multiply/2
  Sqrt/1 -> Multiply/1
  Dot Product/1 -> Divide/1
  Dot Product2/1 -> Sqrt1/1
  Multiply/1 -> Divide/2
  In1/1 -> Dot Product/1
  Gain/1 -> Out1/1

== system Gyro_Outage_Unit_Test/Subsystem5 ==
  Add : Sum
  Eclipse_end : Step  Time=3700.1  After=-1  SampleTime=0
  Eclipse_time : Step  Tag=Eclipse_time  Time=1900  SampleTime=0
  Out1 : Outport
  wires:
  Eclipse_time/1 -> Add/1
  Eclipse_end/1 -> Add/2
  Add/1 -> Out1/1

== system Gyro_Outage_Unit_Test/get Error ==
  q_true : Inport
  q_est : Inport  Port=2
  Quaternion Conjugate : aerolibutil/Quaternion Conjugate
      settings: SourceProductName=Aerospace Blockset  SourceProductBaseCode=AE
  Quaternion Multiplication : aerolibutil/Quaternion Multiplication
  error_quaternion : Outport
  wires:
  Quaternion Conjugate/1 -> Quaternion Multiplication/1
  Quaternion Multiplication/1 -> error_quaternion/1
  q_true/1 -> Quaternion Conjugate/1
  q_est/1 -> Quaternion Multiplication/2

== system Gyro_Outage_Unit_Test/get omega norm ==
  In1 : Inport
  Dot Product : DotProduct  InputSameDT=on  OutDataTypeStr=Inherit: Inherit via internal rule
  Gain : Gain  Gain=180/pi
  Sqrt : Sqrt  SaturateOnIntegerOverflow=on
  Out1 : Outport
  wires:
  Gain/1 -> Out1/1
  Dot Product/1 -> Sqrt/1
  Sqrt/1 -> Gain/1
  In1/1 -> Dot Product/2, Dot Product/1

== system Gyro_Outage_Unit_Test/q_start needed only for certain applications ==
  q_est : Inport
  q_true : Inport  Port=2
  Quaternion Conjugate : aerolibutil/Quaternion Conjugate
      settings: SourceProductName=Aerospace Blockset  SourceProductBaseCode=AE
  Quaternion Multiplication : aerolibutil/Quaternion Multiplication
  error_quaternion : Outport
  wires:
  Quaternion Conjugate/1 -> Quaternion Multiplication/1
  Quaternion Multiplication/1 -> error_quaternion/1
  q_true/1 -> Quaternion Conjugate/1
  q_est/1 -> Quaternion Multiplication/2

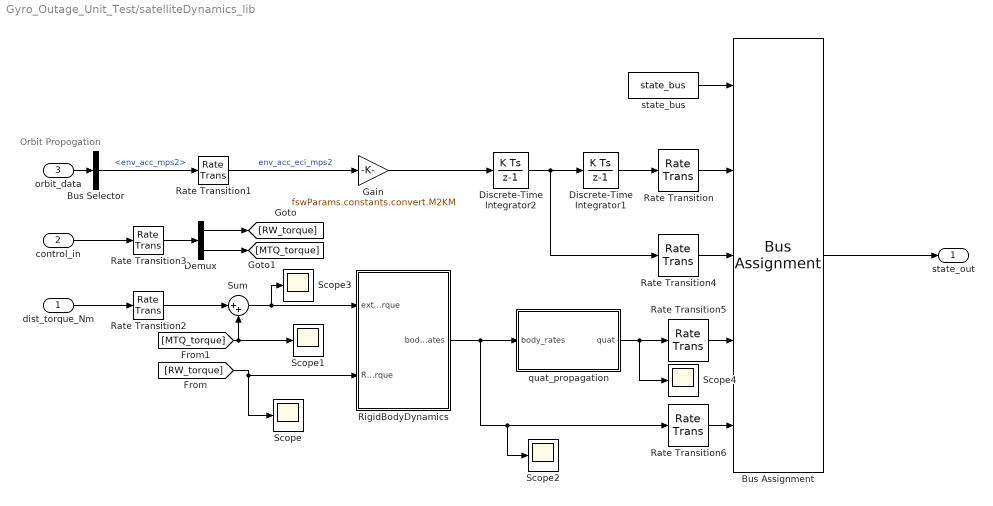
== system Gyro_Outage_Unit_Test/satelliteDynamics_lib ==
  note: Orbit Propogation
  dist_torque_Nm : Inport
  control_in : Inport  Port=2
  orbit_data : Inport  Port=3
  Bus Assignment : BusAssignment  AssignedSignals=r_eci_km,v_eci_km,q_body,w_body_radps
  Bus Selector : BusSelector  OutputSignals=env_acc_mps2
  Demux : Demux  Outputs=[3 3]
  Discrete-Time Integrator1 : DiscreteIntegrator  InitialCondition=simParams.initialConditions.r0  SampleTime=-1  ICPrevOutput=DiscIntNeverNeededParam  ICPrevScaledInput=DiscIntNeverNeededParam
  Discrete-Time Integrator2 : DiscreteIntegrator  InitialCondition=simParams.initialConditions.v0  SampleTime=-1  ICPrevOutput=DiscIntNeverNeededParam  ICPrevScaledInput=DiscIntNeverNeededParam
  Gain : Gain  Gain=fswParams.constants.convert.M2KM
  Rate Transition : RateTransition  InitialCondition=simParams.initialConditions.r0
  Rate Transition1 : RateTransition  OutPortSampleTime=simParams.sample_time_s
  Rate Transition2 : RateTransition  OutPortSampleTime=simParams.sample_time_s
  Rate Transition3 : RateTransition  OutPortSampleTime=simParams.sample_time_s
  Rate Transition4 : RateTransition  InitialCondition=simParams.initialConditions.v0
  Rate Transition5 : RateTransition  InitialCondition=simParams.initialConditions.q0
  Rate Transition6 : RateTransition  InitialCondition=simParams.initialConditions.w0
  RigidBodyDynamics : Subsystem
  Scope{,1..4} (5 alike) : Scope
  Sum : Sum  Inputs=|++
  quat_propagation : Subsystem
  state_bus : state_bus/state_bus  SystemSampleTime=-1
  state_out : Outport
  wires:
  Rate Transition6/1 -> Bus Assignment/5
  Rate Transition5/1 -> Bus Assignment/4
  Rate Transition4/1 -> Bus Assignment/3
  Rate Transition/1 -> Bus Assignment/2
  state_bus/1 -> Bus Assignment/1
  Sum/1 -> Scope3/1, RigidBodyDynamics/1(external_torque)
  [MTQ_torque] -> Sum/2, Scope1/1
  [RW_torque] -> Scope/1, RigidBodyDynamics/2(RW_torque)
  Demux/2 -> [MTQ_torque]
  Demux/1 -> [RW_torque]
  Rate Transition3/1 -> Demux/1
  Rate Transition2/1 -> Sum/1
  RigidBodyDynamics/1(body_rates) -> quat_propagation/1(body_rates), Scope2/1, Rate Transition6/1
  quat_propagation/1(quat) -> Scope4/1, Rate Transition5/1
  Rate Transition1/1 -> Gain/1  "env_acc_eci_mps2"
  dist_torque_Nm/1 -> Rate Transition2/1
  Bus Assignment/1 -> state_out/1
  Gain/1 -> Discrete-Time Integrator2/1
  Discrete-Time Integrator1/1 -> Rate Transition/1
  Discrete-Time Integrator2/1 -> Discrete-Time Integrator1/1, Rate Transition4/1
  control_in/1 -> Rate Transition3/1
  orbit_data/1 -> Bus Selector/1
  Bus Selector/1 -> Rate Transition1/1  "<env_acc_mps2>"

== system Gyro_Outage_Unit_Test/Conversion_lib/sunsensor_body_rad1 ==
  <sunsensor_body_deg> : Inport
  Constant1 : Constant  Value=simParams.sensors.sun_sensor.body2sensor
  Create_Sz : Subsystem
  Demux : Demux  Outputs=2
  Invert 3x3 Matrix : aerolibutil/Invert  3x3 Matrix
  Matrix Multiply : Product
  Matrix Multiply1 : Product
  Mux : Mux  Inputs=3
  Tan : Trigonometry  Operator=tan
  Tan1 : Trigonometry  Operator=tan
  deg2rad : Gain  Gain=pi/180
  need toconvert from sensor to body frame???????? : Product  Multiplication=Matrix(*)
  Out1 : Outport
  wires:
  Tan/1 -> Matrix Multiply/2
  Demux/1 -> Tan1/1, Create_Sz/1(alpha)  "alpha"
  Matrix Multiply/1 -> Mux/2  "sunvec_y"
  Create_Sz/1(Out1) -> Mux/3, Matrix Multiply1/2, Matrix Multiply/1  "sunvec_z"
  Demux/2 -> Tan/1, Create_Sz/2(beta)  "beta"
  Tan1/1 -> Matrix Multiply1/1
  deg2rad/1 -> Demux/1
  Matrix Multiply1/1 -> Mux/1  "sunvec_x"
  <sunsensor_body_deg>/1 -> deg2rad/1
  Constant1/1 -> Invert 3x3 Matrix/1
  Invert 3x3 Matrix/1 -> need toconvert from sensor to body frame????????/1
  Mux/1 -> need toconvert from sensor to body frame????????/2
  need toconvert from sensor to body frame????????/1 -> Out1/1

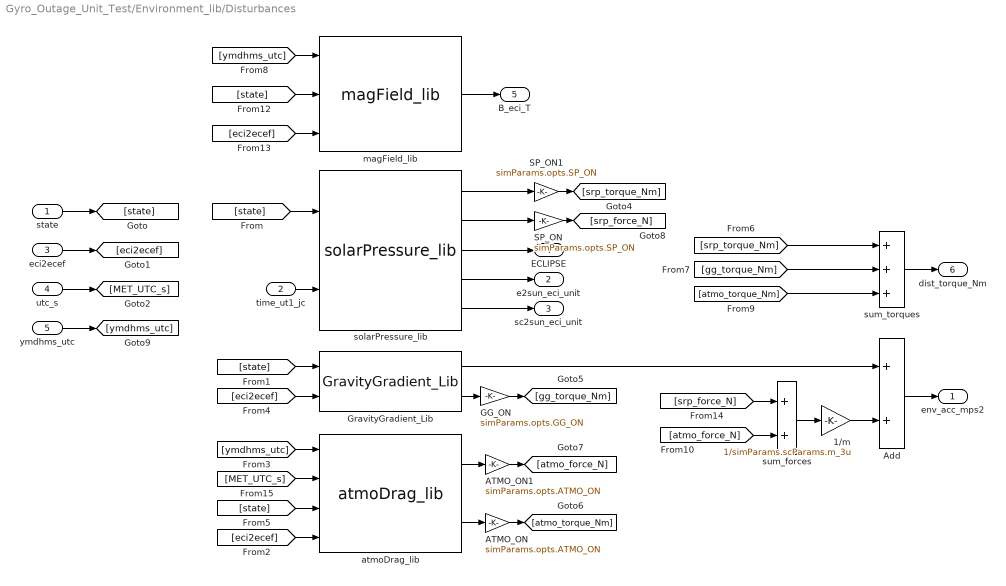
== system Gyro_Outage_Unit_Test/Environment_lib/Disturbances ==
  state : Inport
  time_ut1_jc : Inport  Port=2
  eci2ecef : Inport  Port=3
  utc_s : Inport  Port=4
  ymdhms_utc : Inport  Port=5
  1/m : Gain  Gain=1/simParams.scParams.m_3u
  ATMO_ON : Gain  Gain=simParams.opts.ATMO_ON
  ATMO_ON1 : Gain  Gain=simParams.opts.ATMO_ON
  Add : Sum
  GG_ON : Gain  Gain=simParams.opts.GG_ON
  "GravityGradient_Lib " : gravityGrad_Lib/GravityGradient_Lib   SystemSampleTime=-1
  SP_ON : Gain  Gain=simParams.opts.SP_ON
  "SP_ON1 " : Gain  Gain=simParams.opts.SP_ON
  atmoDrag_lib : atmoDrag_lib/atmoDrag_lib  SystemSampleTime=-1
  magField_lib : magField_lib/magField_lib  SystemSampleTime=-1
      link override Rate Transition2: InitialCondition=0
  solarPressure_lib : solarPressure_lib/solarPressure_lib  SystemSampleTime=-1
  sum_forces : Sum
  sum_torques : Sum  Inputs=+++
  env_acc_mps2 : Outport
  e2sun_eci_unit : Outport  Port=2
  sc2sun_eci_unit : Outport  Port=3
  ECLIPSE : Outport  Port=4
  B_eci_T : Outport  Port=5
  dist_torque_Nm : Outport  Port=6
  wires:
  solarPressure_lib/5 -> sc2sun_eci_unit/1
  magField_lib/1 -> B_eci_T/1
  [eci2ecef] -> magField_lib/3
  [ymdhms_utc] -> magField_lib/1
  ymdhms_utc/1 -> [ymdhms_utc]
  [state] -> magField_lib/2
  "GravityGradient_Lib "/2 -> GG_ON/1
  "GravityGradient_Lib "/1 -> Add/1
  SP_ON/1 -> [srp_force_N]
  ATMO_ON1/1 -> [atmo_force_N]
  [srp_force_N] -> sum_forces/1
  [atmo_force_N] -> sum_forces/2
  [atmo_torque_Nm] -> sum_torques/3
  sum_torques/1 -> dist_torque_Nm/1
  [eci2ecef] -> "GravityGradient_Lib "/2
  [gg_torque_Nm] -> sum_torques/2
  GG_ON/1 -> [gg_torque_Nm]
  [srp_torque_Nm] -> sum_torques/1
  "SP_ON1 "/1 -> [srp_torque_Nm]
  [MET_UTC_s] -> atmoDrag_lib/2
  [ymdhms_utc] -> atmoDrag_lib/1
  utc_s/1 -> [MET_UTC_s]
  [state] -> atmoDrag_lib/3
  [eci2ecef] -> atmoDrag_lib/4
  eci2ecef/1 -> [eci2ecef]
  [state] -> "GravityGradient_Lib "/1
  [state] -> solarPressure_lib/1
  state/1 -> [state]
  ATMO_ON/1 -> [atmo_torque_Nm]
  atmoDrag_lib/1 -> ATMO_ON1/1
  atmoDrag_lib/2 -> ATMO_ON/1
  1/m/1 -> Add/2
  Add/1 -> env_acc_mps2/1
  sum_forces/1 -> 1/m/1
  time_ut1_jc/1 -> solarPressure_lib/2
  solarPressure_lib/2 -> SP_ON/1
  solarPressure_lib/4 -> e2sun_eci_unit/1
  solarPressure_lib/1 -> "SP_ON1 "/1
  solarPressure_lib/3 -> ECLIPSE/1

== system Gyro_Outage_Unit_Test/MEKF_lib1/If Action Subsystem1 ==
  P_chol (-) : Inport
  Bias (-) : Inport  Port=2
  q (-) : Inport  Port=3
  Action Port : ActionPort  ActionType=else
  q (+) : Outport
  P_chol (+) : Outport  Port=2
  Bias (+) : Outport  Port=3
  wires:
  q (-)/1 -> q (+)/1
  Bias (-)/1 -> Bias (+)/1
  P_chol (-)/1 -> P_chol (+)/1

== system Gyro_Outage_Unit_Test/MEKF_lib1/MEKF or Propagation ==
  sun_valid : Inport
  mag_valid : Inport  Port=2
  sun_meas : Inport  Port=3
  mag_meas : Inport  Port=4
  AND : Logic  Inputs=3  AllPortsSameDT=off  OutDataTypeStr=boolean
  Angle_between_vectors : Subsystem  AncestorBlock=MEKF_lib/MEKF_lib/Triad_alg/Triad/Angle_between_vectors
  EKF_Mode : Outport
  wires:
  Angle_between_vectors/1(Parallel_Protection) -> AND/3
  AND/1 -> EKF_Mode/1
  sun_valid/1 -> AND/1
  mag_valid/1 -> AND/2
  sun_meas/1 -> Angle_between_vectors/1(sun_meas_rad_body)
  mag_meas/1 -> Angle_between_vectors/2(mag_meas_T_body)

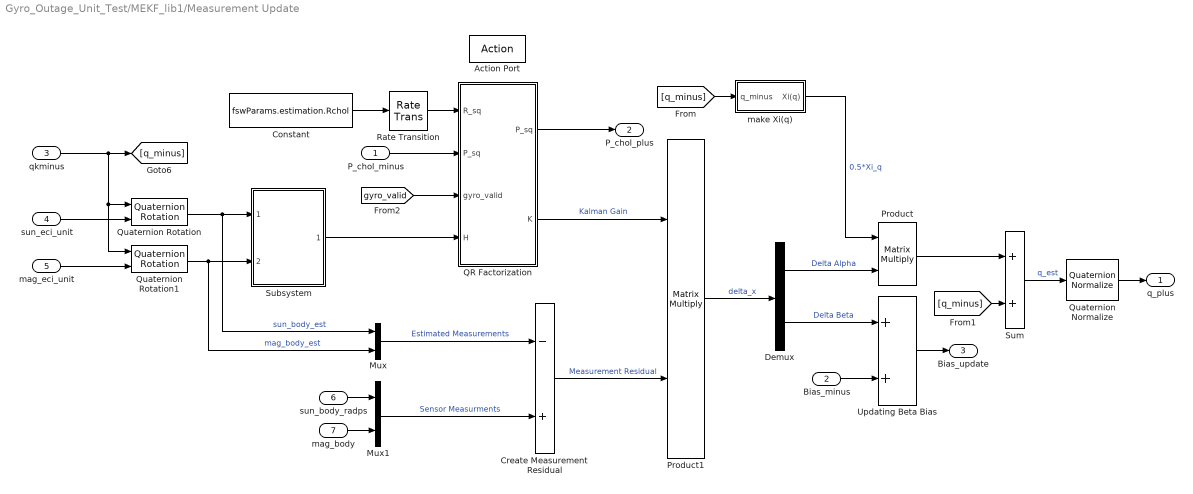
== system Gyro_Outage_Unit_Test/MEKF_lib1/Measurement Update ==
  P_chol_minus : Inport
  Bias_minus : Inport  Port=2
  qkminus : Inport  Port=3
  sun_eci_unit : Inport  Port=4
  mag_eci_unit : Inport  Port=5
  sun_body_radps : Inport  Port=6
  mag_body : Inport  Port=7
  Action Port : ActionPort  ActionType=then
  Constant : Constant  Value=fswParams.estimation.Rchol  VectorParams1D=off
  Create Measurement Residual : Sum  Inputs=-+
  Demux : Demux  Outputs=2
  Mux : Mux  Inputs=2
  Mux1 : Mux  Inputs=2
  Product : Product  Inputs=**  Multiplication=Matrix(*)
  Product1 : Product  Multiplication=Matrix(*)
  QR Factorization : MATLAB Function  TreatAsAtomicUnit=on
  Quaternion Normalize : sharedutil/Quaternion Normalize  aMode=aMode
      settings: SourceProductName=Aerospace Blockset  SourceProductBaseCode=AE
  Quaternion Rotation : aerolibutil/Quaternion Rotation
  Quaternion Rotation1 : aerolibutil/Quaternion Rotation
  Rate Transition : RateTransition  InitialCondition=fswParams.estimation.ic.Rchol_rt  OutPortSampleTime=fswParams.sample_time_s
  Subsystem : Subsystem
  Sum : Sum
  "Updating Beta Bias " : Sum
  make Xi(q) : Subsystem
  q_plus : Outport
  P_chol_plus : Outport  Port=2
  Bias_update : Outport  Port=3
  wires:
  [q_minus] -> Sum/2
  Mux1/1 -> Create Measurement Residual/2  "Sensor Measurments"
  Demux/2 -> "Updating Beta Bias "/1  "Delta Beta"
  Mux/1 -> Create Measurement Residual/1  "Estimated Measurements"
  Bias_minus/1 -> "Updating Beta Bias "/2
  Sum/1 -> Quaternion Normalize/1  "q_est"
  Product/1 -> Sum/1
  Product1/1 -> Demux/1  "delta_x"
  Demux/1 -> Product/2  "Delta Alpha"
  make Xi(q)/1(Xi(q)) -> Product/1  "0.5*Xi_q"
  Quaternion Normalize/1 -> q_plus/1
  Create Measurement Residual/1 -> Product1/2  "Measurement Residual"
  mag_body/1 -> Mux1/2
  sun_body_radps/1 -> Mux1/1
  "Updating Beta Bias "/1 -> Bias_update/1
  sun_eci_unit/1 -> Quaternion Rotation/2
  mag_eci_unit/1 -> Quaternion Rotation1/2
  Quaternion Rotation1/1 -> Subsystem/2(mag_body_hat), Mux/2  "mag_body_est"
  Quaternion Rotation/1 -> Subsystem/1(sun_body_hat), Mux/1  "sun_body_est"
  qkminus/1 -> Quaternion Rotation1/1, Quaternion Rotation/1, [q_minus]
  [q_minus] -> make Xi(q)/1(q_minus)
  Constant/1 -> Rate Transition/1
  P_chol_minus/1 -> QR Factorization/2("P_sq ")
  [gyro_valid] -> QR Factorization/3(gyro_valid)
  Subsystem/1(H_matrix) -> QR Factorization/4(H)
  QR Factorization/1(P_sq) -> P_chol_plus/1
  QR Factorization/2(K) -> Product1/1  "Kalman Gain"
  Rate Transition/1 -> QR Factorization/1(R_sq)

== system Gyro_Outage_Unit_Test/MEKF_lib1/Subsystem ==
  q_k : Inport
  Triad_q : Inport  Port=2
  If Action Subsystem2 : Subsystem  TreatAsAtomicUnit=on
  Unit Delay2 : UnitDelay  InitialCondition=fswParams.estimation.ic.quat_est_init  SampleTime=fswParams.sample_time_s
  Triad_qest : Outport
  q_ekf : Outport  Port=2
  Output : Outport  Port=3
  wires:
  Unit Delay2/1 -> Output/1, If Action Subsystem2/1(In1)
  [Do_MEKF] -> If Action Subsystem2/Action
  q_k/1 -> Unit Delay2/1
  If Action Subsystem2/1(Out1) -> q_ekf/1
  Triad_q/1 -> Triad_qest/1

== system Gyro_Outage_Unit_Test/MEKF_lib1/Three_sigma ==
  P_plus : Inport
  Abs : Abs
  Demux : Demux  Outputs=2
  Extract Diagonal : S-Function  FunctionName=sdspdiag2  Parameters=mode  SFunctionDeploymentMode=off  EnableBusSupport=off  mask(Extract Diagonal){}
      mask help: Extract the main diagonal of a full matrix.
      mask init:
      | mode = 2;
      | x = [.58 .87 NaN 0.12 0.45 0.45 0.12 0.12 NaN 0.525 0.525 0.475 0.475 0.525 0.525 0.565 0.525 ];
      | y = [ 0.8 0.2 NaN 0.2 0.2 0.8 0.8 0.2 NaN 0.435 0.475 0.475 0.525 0.525 0.565 0.5 0.435 ];
      mask Help: eval('blocksethelp');
      mask Display:
      | plot(x,y);
      | port_label('input',1,'A');
      | port_label('output',1,'D');
  Multiply : Gain  Gain=3*180/pi
  Terminator : Terminator
  3Sigma_deg : Outport
  wires:
  Multiply/1 -> 3Sigma_deg/1
  P_plus/1 -> Extract Diagonal/1
  Abs/1 -> Multiply/1
  Extract Diagonal/1 -> Demux/1
  Demux/1 -> Abs/1
  Demux/2 -> Terminator/1
